simulink model "Copy_of_regionprop_test"  (R2015b)
settings: Solver=VariableStepAuto  StartTime=0.0  StopTime=10.0  RelTol=1e-3
values from neighbouring files (symbols this model uses):
  C = img(max(r2+(c1-1)*sx,1))    [IntegralImage_BoxIntegral_mine.m]
undefined symbols (not defined in the file or in its folder): IsPositionTracked, IsSkeletonTracked, JointDepthIndices, JointImageIndices, JointTrackingState, JointWorldCoordinates, PositionDepthIndices, PositionImageIndices, PositionWorldCoordinates, SegmentationData, SkeletonTrackingID, videoinput
libraries: visionsinks x2, visionstatistics x1, imaqlib x1
(part 1 of 11)
settings Model: Creator=FLM  LastModifiedBy=FLM

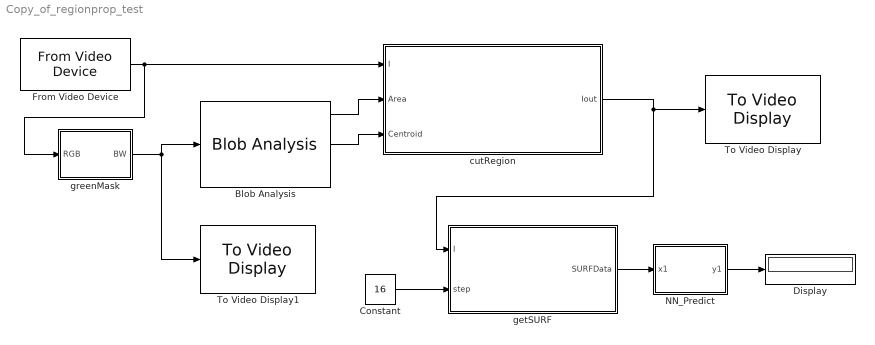
== system Copy_of_regionprop_test ==
  Blob Analysis : visionstatistics/Blob Analysis  Tag=vipblks_row_conv  area=on  centroid=on  bBox=on  majorAxis=off  minorAxis=off  angle=off  eccentricity=off  equivDiameterSq=off  extent=off  perimeter=off  maxBlobs=10  warnIfNumBlobsExceeded=on  isCount=off  useMinArea=off  minArea=0  useMaxArea=off  maxArea=intmax('uint32')  excludeBorderBlob=off  outDT=double  isOutVarDim=off  isFill=on  fillValues=-1  conn=8  isLabel=off  outputMode=Binary point scaling  outputWordLength=32  outputFracLength=16  firstCoeffMode=Binary point scaling  firstCoeffWordLength=16  firstCoeffFracLength=14  secondCoeffMode=Binary point scaling  secondCoeffWordLength=32  secondCoeffFracLength=16  accumMode=Binary point scaling  accumWordLength=32  accumFracLength=0  prodOutputMode=Binary point scaling  prodOutputWordLength=32  prodOutputFracLength=16  roundingMode=Floor  overflowMode=off
  Constant : Constant  Value=16
  Display : Display
  From Video Device : imaqlib/From Video Device  DeviceMenu=winvideo 1 (Integrated Camera)  Device=winvideo 1 (Microsoft? LifeCam Cinema(TM))  ObjConstructor=videoinput('winvideo', 1)  VideoFormatMenu=MJPG_1280x800  VideoFormat=MJPG_320x240  VideoSource=input1  ROIPosition=[0 0 240 320]  EnableHWTrigger=off  SampleTime=1/30  OutputPortsMode=One multidimensional signal  DataType=single  CanDoHWTrigger=no  ReturnedColorSpace=rgb  BlockHandle=1970.0024  ROIWidth=320  ROIHeight=240  ROIColumn=0  ROIRow=0  EngXMLPath=C:\Program Files\MATLAB\R2015b\toolbox\imaq\imaq\private  DevXMLPath=C:\MATLAB\SupportPackages\R2015b\osgenericvideointerface\toolbox\imaq\supportpackages\genericvideo\adaptor\win64  EngLibPath=C:\Program Files\MATLAB\R2015b\toolbox\imaq\imaqblks\imaqmex\win64  ColorSpace=rgb  BayerSensorAlignment=grbg  AllMetadata=IsPositionTracked;IsSkeletonTracked;JointDepthIndices;JointImageIndices;JointTrackingState;JointWorldCoordinates;PositionDepthIndices;PositionImageIndices;PositionWorldCoordinates;SegmentationData;SkeletonTrackingID
  NN_Predict : MATLAB Function  TreatAsAtomicUnit=on
  To Video Display : visionsinks/To Video Display  windowSizeMode=Normal  openAtMdlStart=on  fullScreen=off  videoWindowX=536805376  videoWindowY=536805376  saveWindowSize=off  videoWindowWidth=160  videoWindowHeight=160  inputColorFormat=RGB  inputType=Obsolete  imagePorts=One multidimensional signal  OutputDevice=On-screen video monitor  dataOrg=Column-major  isWindowOpen=off
  To Video Display1 : visionsinks/To Video Display  windowSizeMode=Normal  openAtMdlStart=on  fullScreen=off  videoWindowX=536805376  videoWindowY=536805376  saveWindowSize=off  videoWindowWidth=160  videoWindowHeight=160  inputColorFormat=RGB  inputType=Obsolete  imagePorts=One multidimensional signal  OutputDevice=On-screen video monitor  dataOrg=Column-major  isWindowOpen=off
  cutRegion : MATLAB Function  TreatAsAtomicUnit=on
  getSURF : MATLAB Function  TreatAsAtomicUnit=on
  greenMask : MATLAB Function  TreatAsAtomicUnit=on
  wires:
  greenMask/1(BW) -> To Video Display1/1, Blob Analysis/1
  Blob Analysis/2 -> cutRegion/3(Centroid)
  Blob Analysis/1 -> cutRegion/2(Area)
  From Video Device/1 -> greenMask/1(RGB), cutRegion/1(I)
  Constant/1 -> getSURF/2(step)
  getSURF/1(SURFData) -> NN_Predict/1(x1)
  NN_Predict/1(y1) -> Display/1
  cutRegion/1(Iout) -> getSURF/1(I), To Video Display/1

== matlab function Copy_of_regionprop_test/cutRegion ==
  data: I input size=[240,320,3]; Area input; Centroid input; Iout output size=[160,160,3]
function Iout   = cutRegion(I,Area,Centroid)
%#codegen
[Asort,index] = sort(Area,'descend');
cutSize = 160;
translation = [0,-20]; %move up 20 pixel
if Asort(1)<1000
    x = size(I,2)/2;
    y = size(I,1)/2;
else
    index = index(1);
    
    x = Centroid(index,1);
    y = Centroid(index,2);
end
x=round(x); y=round(y);
left =x-cutSize/2 + translation(1)+1;
right = x+cutSize/2 + translation(1);
top = y-cutSize/2 + translation(2)+1;
bottom = y+cutSize/2 + translation(2);
if left<1
    left = 1; right = cutSize;
end
if right>size(I,2)
    right = size(I,2);
    left = right - cutSize + 1;
end
if top < 1
    top = 1; bottom = cutSize;
end
if bottom > size(I,1)
    bottom = size(I,1);
    top = bottom - cutSize+1;
end
Iout=I(top:bottom,left:right,1:3);
end

== matlab function Copy_of_regionprop_test/greenMask ==
  data: RGB input; BW output
function BW = greenMask(RGB)
%#codegen

%function [BW,maskedRGBImage] = createMask5(RGB)
%createMask  Threshold RGB image using auto-generated code from colorThresholder app.
%  [BW,MASKEDRGBIMAGE] = createMask(RGB) thresholds image RGB using
%  auto-generated code from the colorThresholder App. The colorspace and
%  minimum/maximum values for each channel of the colorspace were set in the
%  App and result in a binary mask BW and a composite image maskedRGBImage,
%  which shows the original RGB image values under the mask BW.

% Auto-generated by colorThresholder app on 01-Mar-2016
%------------------------------------------------------


% Convert RGB image to chosen color space
I = rgb2hsv(RGB);

% Define thresholds for channel 1 based on histogram settings
channel1Min = 0.187;
channel1Max = 0.514;

% Define thresholds for channel 2 based on histogram settings
channel2Min = 0.196;
channel2Max = 1.000;

% Define thresholds for channel 3 based on histogram settings
channel3Min = 0.000;
channel3Max = 0.650;

% Create mask based on chosen histogram thresholds
BW = (I(:,:,1) >= channel1Min ) & (I(:,:,1) <= channel1Max) & ...
    (I(:,:,2) >= channel2Min ) & (I(:,:,2) <= channel2Max) & ...
    (I(:,:,3) >= channel3Min ) & (I(:,:,3) <= channel3Max);

% Initialize output masked image based on input image.
%maskedRGBImage = RGB;

% Set background pixels where BW is false to zero.
%maskedRGBImage(repmat(~BW,[1 1 3])) = 0;

== matlab function Copy_of_regionprop_test/getSURF ==
  data: I input; SURFData output; step input
function SURFData   = getSURF_surf( I,step )
%#codegen
SURFData = getSURF_surf(I,step);
end
